simulink model "DynamicVibration"  (R2020b)
settings: Solver=VariableStepAuto  StartTime=0.0  StopTime=10  RelTol=1e-3
model workspace (MAT data in the model file):
  M1 = 100
  M2 = 2
  b = 50
  k1 = 50
  k2 = 1
settings Model: Creator=DELL  LastModifiedBy=DELL

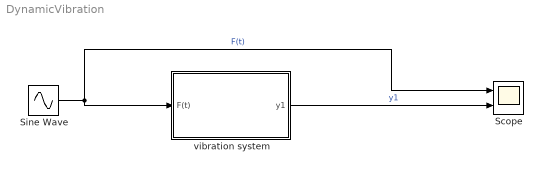
== system DynamicVibration ==
  Scope : Scope  NumInputPorts=2
  Sine Wave : Sin  Amplitude=2  Frequency=10  SampleTime=0
  vibration system : Subsystem
  wires:
  Sine Wave/1 -> vibration system/1(F(t)), Scope/1  "F(t)"
  vibration system/1(y1) -> Scope/2  "y1"

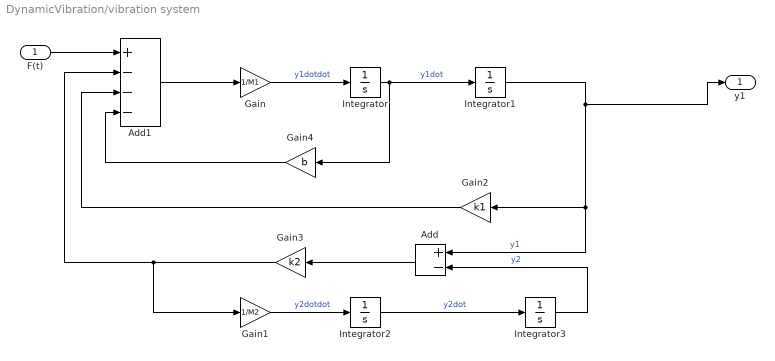
== system DynamicVibration/vibration system ==
  F(t) : Inport
  Add : Sum  Inputs=+-
  Add1 : Sum  Inputs=+---
  Gain : Gain  Gain=1/M1
  Gain1 : Gain  Gain=1/M2
  Gain2 : Gain  Gain=k1
  Gain3 : Gain  Gain=k2
  Gain4 : Gain  Gain=b
  Integrator{,1..3} (4 alike) : Integrator
  y1 : Outport
  wires:
  Add/1 -> Gain3/1
  Integrator2/1 -> Integrator3/1  "y2dot"
  Gain4/1 -> Add1/4
  Add1/1 -> Gain/1
  Integrator/1 -> Gain4/1, Integrator1/1  "y1dot"
  Gain3/1 -> Gain1/1, Add1/2
  Gain1/1 -> Integrator2/1  "y2dotdot"
  Integrator1/1 -> y1/1, Gain2/1, Add/1  "y1"
  Gain/1 -> Integrator/1  "y1dotdot"
  Gain2/1 -> Add1/3
  Integrator3/1 -> Add/2  "y2"
  F(t)/1 -> Add1/1
